simulink model "req15"  (R2019a)
settings: Solver=FixedStepAuto  StartTime=0.0  StopTime=100  RelTol=1e-3
libraries: simulink x1
settings Model: Creator=e40014285  LastModifiedBy=e40014285
settings ConfigComp: CovScope=ReferencedModels  CovHTMLOptions=-sRT=1 -sVT=0 -aTS=1 -bRG=1 -bTC=1 -hTR=0 -nFC=0 -nFD=1 -scm=1 -bcm=1 -xEv=0 -xEM=0  CovHtmlReporting=on  CovCumulativeReport=on  DVModelCoverageObjectives=EnhancedMCDC  DVTestSuiteOptimization=Auto  DVDetectOutOfBounds=on  DVReportPDFFormat=on  DVRebuildModelRepresentation=Always

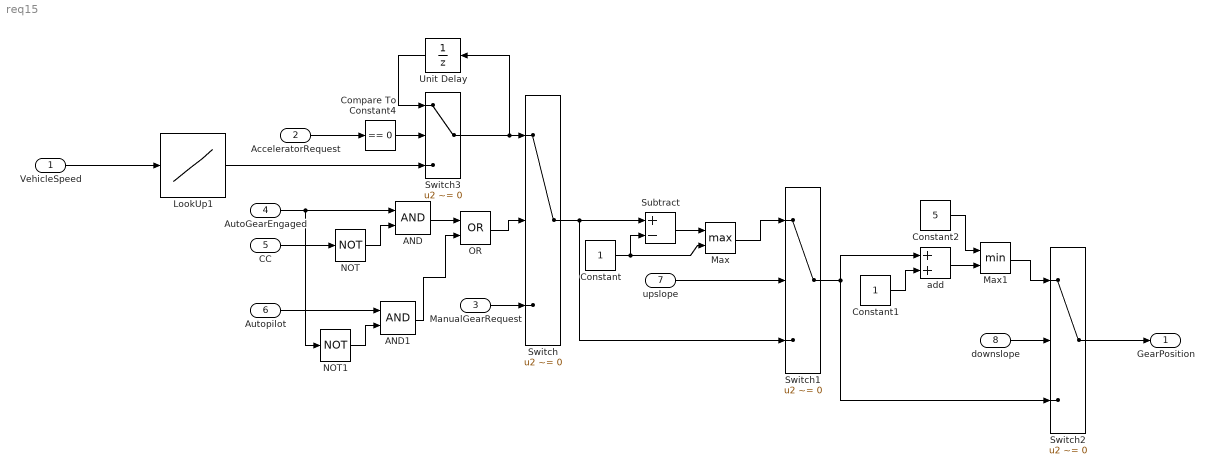
== system req15 ==
  VehicleSpeed : Inport
  AcceleratorRequest : Inport  Port=2
  ManualGearRequest : Inport  Port=3
  AutoGearEngaged : Inport  Port=4
  CC : Inport  Port=5
  Autopilot : Inport  Port=6
  upslope : Inport  Port=7
  downslope : Inport  Port=8
  AND : Logic  AllPortsSameDT=off  OutDataTypeStr=boolean
  AND1 : Logic  AllPortsSameDT=off  OutDataTypeStr=boolean
  Compare To Constant4 : simulink/Logic and Bit Operations/Compare To Constant  relop===  const=0  OutDataTypeStr=boolean
  Constant : Constant
  Constant1 : Constant
  Constant2 : Constant  Value=5
  LookUp1 : Lookup_n-D  NumberOfTableDimensions=1  BreakpointsForDimension1=[0 20 30 40 60]  Table=[1 2 3 4 5]  InterpMethod=Flat  RemoveProtectionInput=on  InternalRulePriority=Speed  RndMeth=Simplest  InputSameDT=on
  Max : MinMax  Function=max  Inputs=2
  Max1 : MinMax  Inputs=2
  NOT : Logic  Operator=NOT  AllPortsSameDT=off  OutDataTypeStr=boolean
  NOT1 : Logic  Operator=NOT  AllPortsSameDT=off  OutDataTypeStr=boolean
  OR : Logic  Operator=OR  AllPortsSameDT=off  OutDataTypeStr=boolean
  Subtract : Sum  Inputs=+-
  Switch{,1..3} (4 alike) : Switch  Criteria=u2 ~= 0
  Unit Delay : UnitDelay  SampleTime=-1  HasFrameUpgradeWarning=on
  add : Sum
  GearPosition : Outport
  wires:
  Switch/1 -> Switch1/3, Subtract/1
  ManualGearRequest/1 -> Switch/3
  AutoGearEngaged/1 -> AND/1, NOT1/1
  Compare To Constant4/1 -> Switch3/2
  Switch3/1 -> Switch/1, Unit Delay/1
  Unit Delay/1 -> Switch3/1
  AcceleratorRequest/1 -> Compare To Constant4/1
  VehicleSpeed/1 -> LookUp1/1
  LookUp1/1 -> Switch3/3
  CC/1 -> NOT/1
  NOT/1 -> AND/2
  AND/1 -> OR/1
  OR/1 -> Switch/2
  NOT1/1 -> AND1/2
  Autopilot/1 -> AND1/1
  AND1/1 -> OR/2
  upslope/1 -> Switch1/2
  Constant/1 -> Max/2, Subtract/2
  Subtract/1 -> Max/1
  Max/1 -> Switch1/1
  downslope/1 -> Switch2/2
  Switch1/1 -> Switch2/3, add/1
  Constant1/1 -> add/2
  add/1 -> Max1/2
  Constant2/1 -> Max1/1
  Max1/1 -> Switch2/1
  Switch2/1 -> GearPosition/1
